simulink model "System"  (R2014b)
settings: Solver=ode45  StartTime=0.0  StopTime=20  FixedStep=0.05  RelTol=1e-3
PreLoadFcn:
  | Init
model workspace (MAT data in the model file):
  InitPose = Simulink.Parameter
  InitPose.Value = 0.14112000806
  InitPose.DataType = 'auto'
libraries: roblocks x5, lib x2, dspinverses x1, dspmtrx3 x1, simulink x1
settings Model: NumberOfSteps=50  ExtModeTrigMode=oneshot  ExtModeArmWhenConnect=off  Creator=pic  LastModifiedBy=Edoardo
settings DataIOCC: LimitDataPoints=off  SignalLogging=off  ReturnWorkspaceOutputs=on
settings OptimizationCC: BlockReduction=off  BooleanDataType=off  ExpressionDepthLimit=2147483647  InitFltsAndDblsToZero=on
settings DebuggingCC: SaveWithParameterizedLinksMsg=none  SignalResolutionControl=TryResolveAllWithWarning  SolverPrmCheckMsg=none  MultiTaskDSMMsg=warning  MultiTaskCondExecSysMsg=none  FcnCallInpInsideContextMsg=UseLocalSettings  StateNameClashWarn=warning
settings HardwareCC: TargetUnknown=on
settings ModelReferenceCC: ModelReferenceNumInstancesAllowed=Single
settings RTWCC: IncludeERTFirstTime=on
settings GRTTargetCC: ModelReferenceCompliant=off  CompOptLevelCompliant=off  CombineOutputUpdateFcns=off  MatFileLogging=off  GRTInterface=on

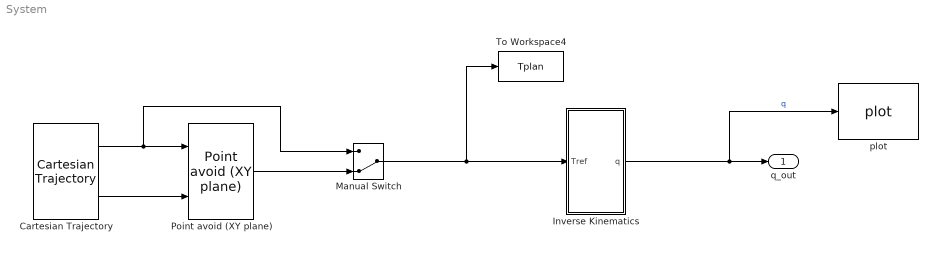
== system System ==
  "Cartesian Trajectory " : lib/Cartesian  Trajectory  ref=Internal  T0=T0  Tf=T0  v={T4}  Tmax=20  Ts=0.1
  Inverse Kinematics : Subsystem  mask{Jd=0, K=5}
      mask prompts: Jd "Jacobian damping"; K "Error gain"
  Manual Switch : ManualSwitch  CurrentSetting=0
  Point avoid (XY plane) : lib/Point avoid (XY plane)  pt=[0 0 0]  r=0.4
  To Workspace4 : ToWorkspace  VariableName=Tplan  SampleTime=-1
  plot : roblocks/Robot Graphics/plot  robot=robot  fps=25  holdplot=on
  q_out : Outport
  wires:
  Manual Switch/1 -> Inverse Kinematics/1(Tref), To Workspace4/1
  Point avoid (XY plane)/1 -> Manual Switch/2
  Inverse Kinematics/1(q) -> q_out/1, plot/1  "q"
  "Cartesian Trajectory "/1 -> Point avoid (XY plane)/1, Manual Switch/1
  "Cartesian Trajectory "/2 -> Point avoid (XY plane)/2

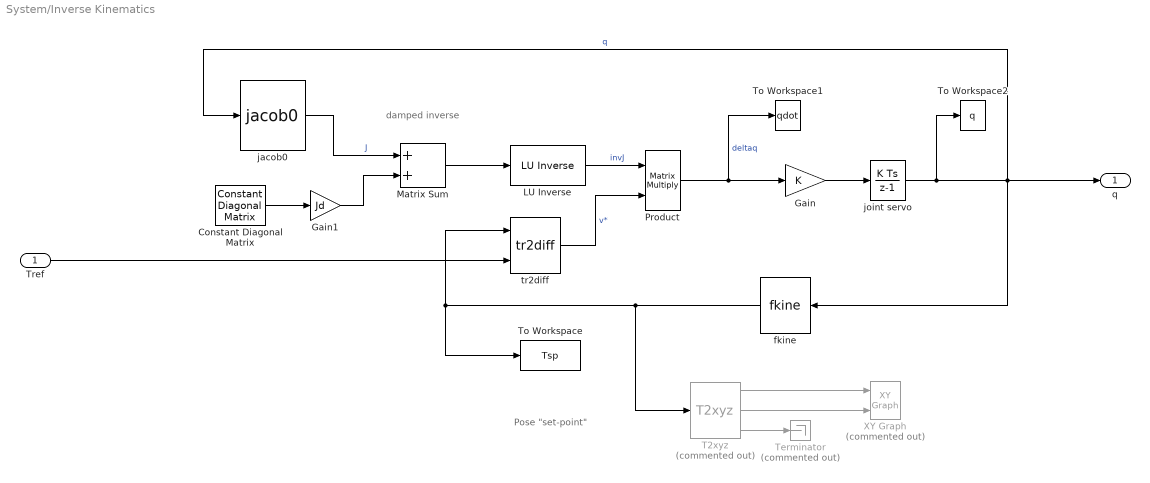
== system System/Inverse Kinematics ==
  note: Pose "set-point"
  note: damped inverse
  Tref : Inport
  " LU Inverse" : dspinverses/ LU Inverse
  Constant Diagonal Matrix : dspmtrx3/Constant Diagonal Matrix  q=ones(1,6)  frame=off  dataType=Inherit from 'Constant(s) along diagonal'  isSigned=on  wordLen=16  udDataType=sfix(16)  fracBitsMode=Best precision  numFracBits=15
  Gain : Gain  Gain=K  SaturateOnIntegerOverflow=on  OutDataTypeStr=Inherit: Same as input  ParamDataTypeStr=Inherit: Same as input
  Gain1 : Gain  Gain=Jd
  Matrix Sum : Sum
  Product : Product  Multiplication=Matrix(*)  SaturateOnIntegerOverflow=on  RndMeth=Zero  InputSameDT=on  OutDataTypeStr=Inherit: Same as first input
  T2xyz : roblocks/Transform Conversion/T2xyz  Commented=on
  Terminator : Terminator  Commented=on
  To Workspace : ToWorkspace  VariableName=Tsp  SampleTime=-1
  To Workspace1 : ToWorkspace  VariableName=qdot  SampleTime=-1
  To Workspace2 : ToWorkspace  VariableName=q  SampleTime=-1
  XY Graph : simulink/Sinks/XY Graph  Commented=on  xmin=-1  xmax=1  ymin=-1  ymax=1  st=-1
  fkine : roblocks/Kinematics/fkine  robot=robot
  "jacob0 " : roblocks/Kinematics/jacob0   robot=robot
  joint servo : DiscreteIntegrator  InitialCondition=qn'  SampleTime=0.05
  tr2diff : roblocks/Kinematics/tr2diff  robot=robot
  q : Outport
  wires:
  Constant Diagonal Matrix/1 -> Gain1/1
  Gain/1 -> joint servo/1
  " LU Inverse"/1 -> Product/1  "invJ"
  fkine/1 -> T2xyz/1, To Workspace/1, tr2diff/1
  Tref/1 -> tr2diff/2
  T2xyz/1 -> XY Graph/1
  Gain1/1 -> Matrix Sum/2
  "jacob0 "/1 -> Matrix Sum/1  "J"
  tr2diff/1 -> Product/2  "v*"
  T2xyz/2 -> XY Graph/2
  Matrix Sum/1 -> " LU Inverse"/1
  Product/1 -> To Workspace1/1, Gain/1  "deltaq"
  T2xyz/3 -> Terminator/1
  joint servo/1 -> To Workspace2/1, q/1, "jacob0 "/1, fkine/1  "q"
